simulink model "aocs_plant_pre_high_accuracy_eci_ecef"  (R2025a)
settings: Solver=ode45  StartTime=0  StopTime=200  RelTol=1e-09  AbsTol=1e-10
undefined symbols (not defined in the file): AOCS, AOCS_Config, AOCS_EnvironmentConfig, AOCS_OrbitConfig, IAU, juliandate
libraries: aerolibtransform2 x3, matrix_library x1
settings Model: Creator=juliankazmierski  LastModifiedBy=juliankazmierski

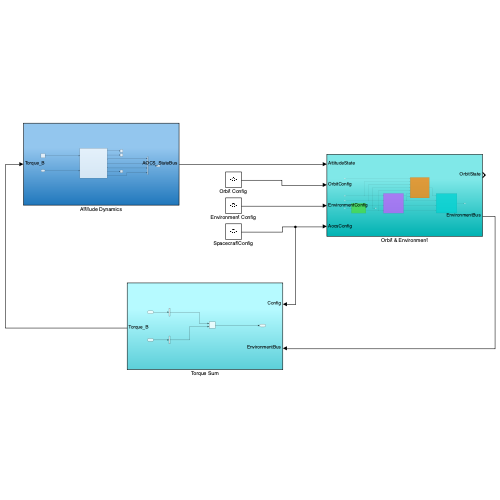
[thumbnail: Simulink's stored preview of the top-level diagram]
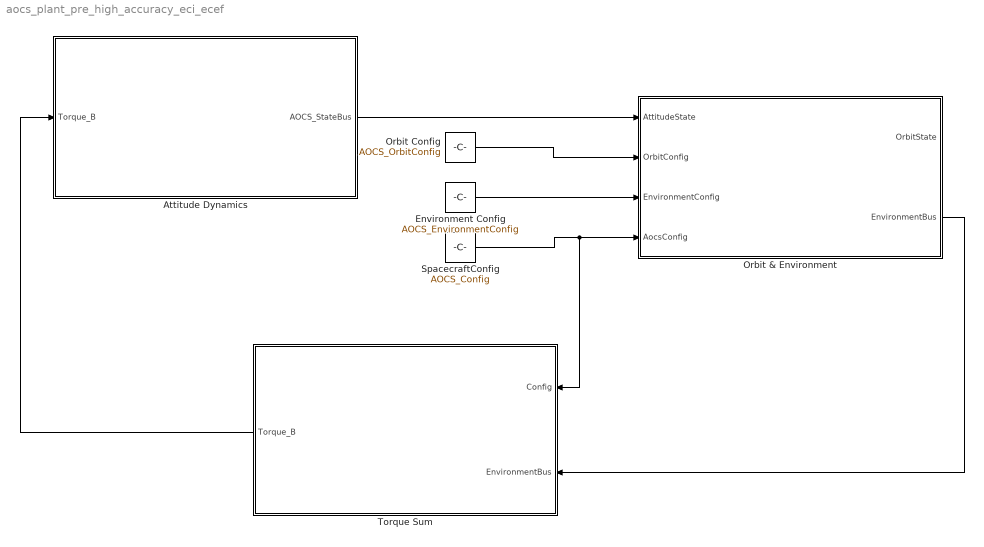
== system aocs_plant_pre_high_accuracy_eci_ecef ==
  Attitude Dynamics : Subsystem
  Environment Config : Constant  Value=AOCS_EnvironmentConfig  OutDataTypeStr=Bus: AOCS_EnvironmentConfigBus
  Orbit & Environment : Subsystem
  Orbit Config : Constant  Value=AOCS_OrbitConfig  VectorParams1D=off  OutDataTypeStr=Bus: AOCS_OrbitConfigBus
  SpacecraftConfig : Constant  Value=AOCS_Config  OutDataTypeStr=Bus: AOCS_ConfigBus
  Torque Sum : Subsystem
  wires:
  SpacecraftConfig/1 -> Orbit & Environment/4(AocsConfig), Torque Sum/1(Config)
  Attitude Dynamics/1(AOCS_StateBus) -> Orbit & Environment/1(AttitudeState)
  Orbit Config/1 -> Orbit & Environment/2(OrbitConfig)
  Environment Config/1 -> Orbit & Environment/3(EnvironmentConfig)
  Orbit & Environment/2(EnvironmentBus) -> Torque Sum/2(EnvironmentBus)
  Torque Sum/1(Torque_B) -> Attitude Dynamics/1(Torque_B)

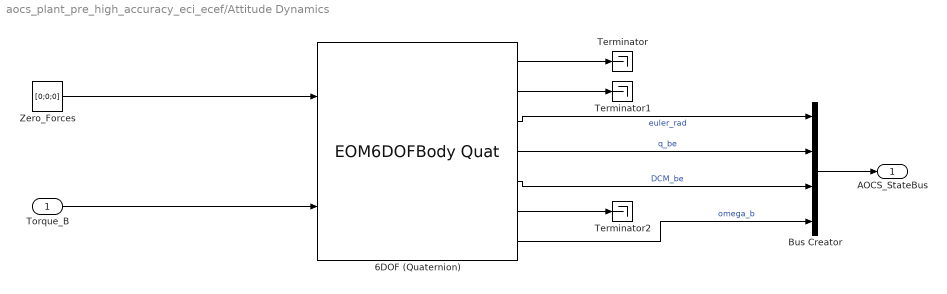
== system aocs_plant_pre_high_accuracy_eci_ecef/Attitude Dynamics ==
  Torque_B : Inport
  6DOF (Quaternion) : EOM6DOFBodyQuat  eul_0=AOCS_Config.euler_BI_0_rad  pm_0=AOCS_Config.omega_BI_B_0  mass_0=3.71  inertia=AOCS_Config.I_B
  Bus Creator : BusCreator  Inputs=4
  Terminator : Terminator
  Terminator1 : Terminator
  Terminator2 : Terminator
  Zero_Forces : Constant  Value=[0;0;0]
  AOCS_StateBus : Outport  OutDataTypeStr=Bus: AOCS_StateBus
  wires:
  Torque_B/1 -> 6DOF (Quaternion)/2
  Zero_Forces/1 -> 6DOF (Quaternion)/1
  6DOF (Quaternion)/1 -> Terminator/1
  6DOF (Quaternion)/2 -> Terminator1/1
  6DOF (Quaternion)/6 -> Terminator2/1
  6DOF (Quaternion)/3 -> Bus Creator/1  "euler_rad"
  6DOF (Quaternion)/5 -> Bus Creator/3  "DCM_be"
  6DOF (Quaternion)/7 -> Bus Creator/4  "omega_b"
  Bus Creator/1 -> AOCS_StateBus/1
  6DOF (Quaternion)/4 -> Bus Creator/2  "q_be"

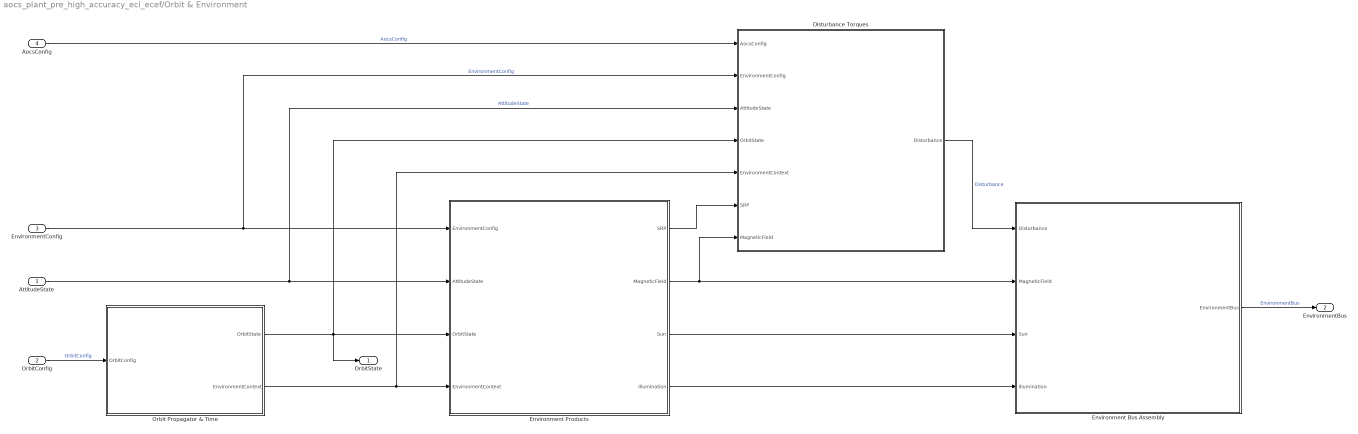
== system aocs_plant_pre_high_accuracy_eci_ecef/Orbit & Environment ==
  AttitudeState : Inport
  OrbitConfig : Inport  Port=2
  EnvironmentConfig : Inport  Port=3
  AocsConfig : Inport  Port=4
  Disturbance Torques : Subsystem
  Environment Bus Assembly : Subsystem
  Environment Products : Subsystem
  Orbit Propagator & Time : Subsystem
  OrbitState : Outport  OutDataTypeStr=Bus: AOCS_OrbitStateBus
  EnvironmentBus : Outport  Port=2  OutDataTypeStr=Bus: AOCS_EnvironmentBus
  wires:
  AocsConfig/1 -> Disturbance Torques/1(AocsConfig)  "AocsConfig"
  Disturbance Torques/1(Disturbance) -> Environment Bus Assembly/1(Disturbance)  "Disturbance"
  Environment Bus Assembly/1(EnvironmentBus) -> EnvironmentBus/1  "EnvironmentBus"
  Environment Products/2(MagneticField) -> Disturbance Torques/7(MagneticField), Environment Bus Assembly/2(MagneticField)
  AttitudeState/1 -> Disturbance Torques/3(AttitudeState), Environment Products/2(AttitudeState)  "AttitudeState"
  Orbit Propagator & Time/1(OrbitState) -> OrbitState/1, Disturbance Torques/4(OrbitState), Environment Products/3(OrbitState)
  Orbit Propagator & Time/2(EnvironmentContext) -> Disturbance Torques/5(EnvironmentContext), Environment Products/4(EnvironmentContext)
  EnvironmentConfig/1 -> Environment Products/1(EnvironmentConfig), Disturbance Torques/2(EnvironmentConfig)  "EnvironmentConfig"
  Environment Products/1(SRP) -> Disturbance Torques/6(SRP)
  Environment Products/4(Illumination) -> Environment Bus Assembly/4(Illumination)
  Environment Products/3(Sun) -> Environment Bus Assembly/3(Sun)
  OrbitConfig/1 -> Orbit Propagator & Time/1(OrbitConfig)  "OrbitConfig"

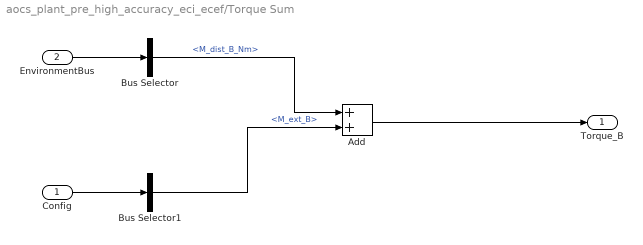
== system aocs_plant_pre_high_accuracy_eci_ecef/Torque Sum ==
  Config : Inport
  EnvironmentBus : Inport  Port=2
  Add : Sum
  Bus Selector : BusSelector  OutputSignals=M_dist_B_Nm
  Bus Selector1 : BusSelector  OutputSignals=M_ext_B
  Torque_B : Outport
  wires:
  EnvironmentBus/1 -> Bus Selector/1
  Bus Selector/1 -> Add/1  "<M_dist_B_Nm>"
  Add/1 -> Torque_B/1
  Config/1 -> Bus Selector1/1
  Bus Selector1/1 -> Add/2  "<M_ext_B>"

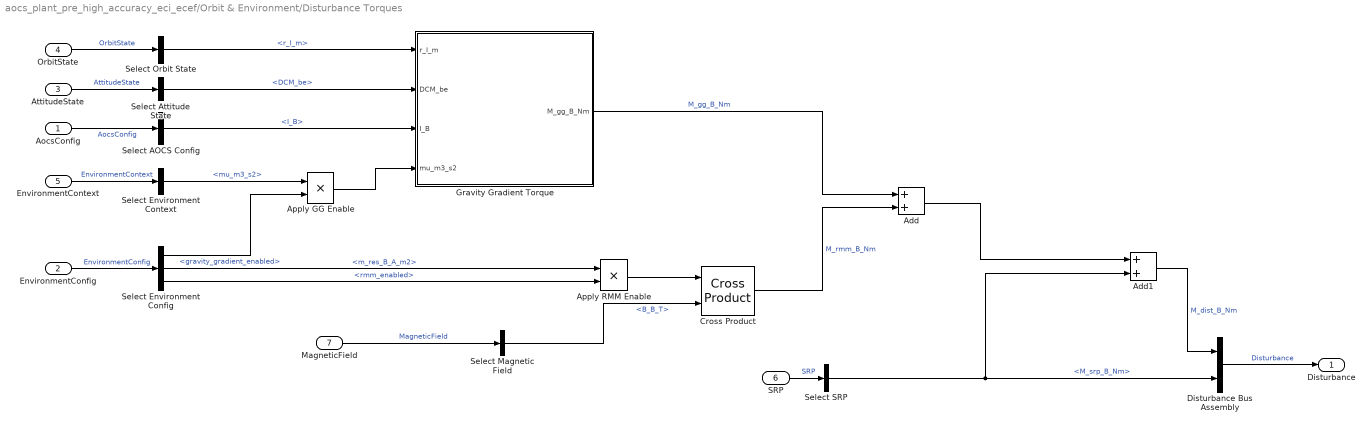
== system aocs_plant_pre_high_accuracy_eci_ecef/Orbit & Environment/Disturbance Torques ==
  AocsConfig : Inport
  EnvironmentConfig : Inport  Port=2
  AttitudeState : Inport  Port=3
  OrbitState : Inport  Port=4
  EnvironmentContext : Inport  Port=5
  SRP : Inport  Port=6
  MagneticField : Inport  Port=7
  Add : Sum
  Add1 : Sum
  Apply GG Enable : Product
  Apply RMM Enable : Product
  Cross Product : matrix_library/Cross Product
  Disturbance Bus Assembly : BusCreator  Inputs=2  OutDataTypeStr=Bus: AOCS_DisturbanceBus
  Gravity Gradient Torque : MATLAB Function  TreatAsAtomicUnit=on
  Select AOCS Config : BusSelector  OutputSignals=I_B
  Select Attitude State : BusSelector  OutputSignals=DCM_be
  Select Environment Config : BusSelector  OutputSignals=gravity_gradient_enabled,m_res_B_A_m2,rmm_enabled
  Select Environment Context : BusSelector  OutputSignals=mu_m3_s2
  Select Magnetic Field : BusSelector  OutputSignals=B_B_T
  Select Orbit State : BusSelector  OutputSignals=r_I_m
  Select SRP : BusSelector  OutputSignals=M_srp_B_Nm
  Disturbance : Outport
  wires:
  Cross Product/1 -> Add/2  "M_rmm_B_Nm"
  Gravity Gradient Torque/1(M_gg_B_Nm) -> Add/1  "M_gg_B_Nm"
  SRP/1 -> Select SRP/1  "SRP"
  Add1/1 -> Disturbance Bus Assembly/1  "M_dist_B_Nm"
  Apply RMM Enable/1 -> Cross Product/1
  Apply GG Enable/1 -> Gravity Gradient Torque/4(mu_m3_s2)
  AocsConfig/1 -> Select AOCS Config/1  "AocsConfig"
  Select AOCS Config/1 -> Gravity Gradient Torque/3(I_B)  "<I_B>"
  EnvironmentConfig/1 -> Select Environment Config/1  "EnvironmentConfig"
  Select Environment Config/2 -> Apply RMM Enable/1  "<m_res_B_A_m2>"
  Select Environment Config/3 -> Apply RMM Enable/2  "<rmm_enabled>"
  Select Environment Config/1 -> Apply GG Enable/2  "<gravity_gradient_enabled>"
  AttitudeState/1 -> Select Attitude State/1  "AttitudeState"
  Select Attitude State/1 -> Gravity Gradient Torque/2(DCM_be)  "<DCM_be>"
  MagneticField/1 -> Select Magnetic Field/1  "MagneticField"
  Select Magnetic Field/1 -> Cross Product/2  "<B_B_T>"
  OrbitState/1 -> Select Orbit State/1  "OrbitState"
  Select Orbit State/1 -> Gravity Gradient Torque/1(r_I_m)  "<r_I_m>"
  EnvironmentContext/1 -> Select Environment Context/1  "EnvironmentContext"
  Select Environment Context/1 -> Apply GG Enable/1  "<mu_m3_s2>"
  Select SRP/1 -> Add1/2, Disturbance Bus Assembly/2  "<M_srp_B_Nm>"
  Disturbance Bus Assembly/1 -> Disturbance/1  "Disturbance"
  Add/1 -> Add1/1

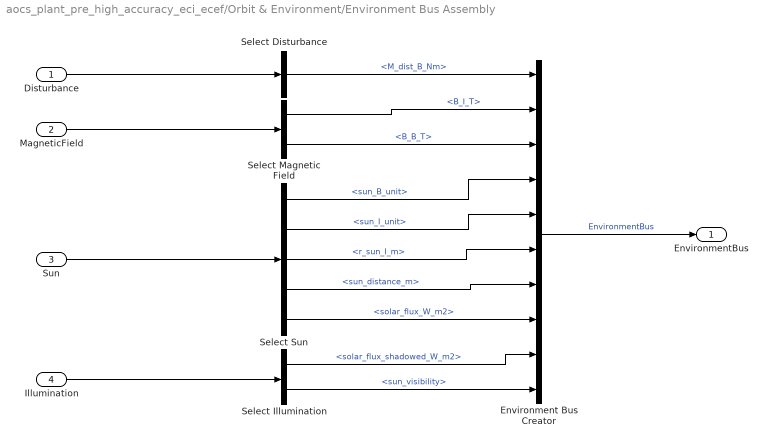
== system aocs_plant_pre_high_accuracy_eci_ecef/Orbit & Environment/Environment Bus Assembly ==
  Disturbance : Inport
  MagneticField : Inport  Port=2
  Sun : Inport  Port=3
  Illumination : Inport  Port=4
  Environment Bus Creator : BusCreator  Inputs=10  OutDataTypeStr=Bus: AOCS_EnvironmentBus
  Select Disturbance : BusSelector  OutputSignals=M_dist_B_Nm
  Select Illumination : BusSelector  OutputSignals=solar_flux_shadowed_W_m2,sun_visibility
  Select Magnetic Field : BusSelector  OutputSignals=B_I_T,B_B_T
  Select Sun : BusSelector  OutputSignals=sun_B_unit,sun_I_unit,r_sun_I_m,sun_distance_m,solar_flux_W_m2
  EnvironmentBus : Outport
  wires:
  Disturbance/1 -> Select Disturbance/1
  Select Disturbance/1 -> Environment Bus Creator/1  "<M_dist_B_Nm>"
  MagneticField/1 -> Select Magnetic Field/1
  Select Magnetic Field/1 -> Environment Bus Creator/2  "<B_I_T>"
  Select Magnetic Field/2 -> Environment Bus Creator/3  "<B_B_T>"
  Sun/1 -> Select Sun/1
  Select Sun/1 -> Environment Bus Creator/4  "<sun_B_unit>"
  Select Sun/2 -> Environment Bus Creator/5  "<sun_I_unit>"
  Select Sun/3 -> Environment Bus Creator/6  "<r_sun_I_m>"
  Select Sun/4 -> Environment Bus Creator/7  "<sun_distance_m>"
  Select Sun/5 -> Environment Bus Creator/8  "<solar_flux_W_m2>"
  Illumination/1 -> Select Illumination/1
  Select Illumination/1 -> Environment Bus Creator/9  "<solar_flux_shadowed_W_m2>"
  Select Illumination/2 -> Environment Bus Creator/10  "<sun_visibility>"
  Environment Bus Creator/1 -> EnvironmentBus/1  "EnvironmentBus"

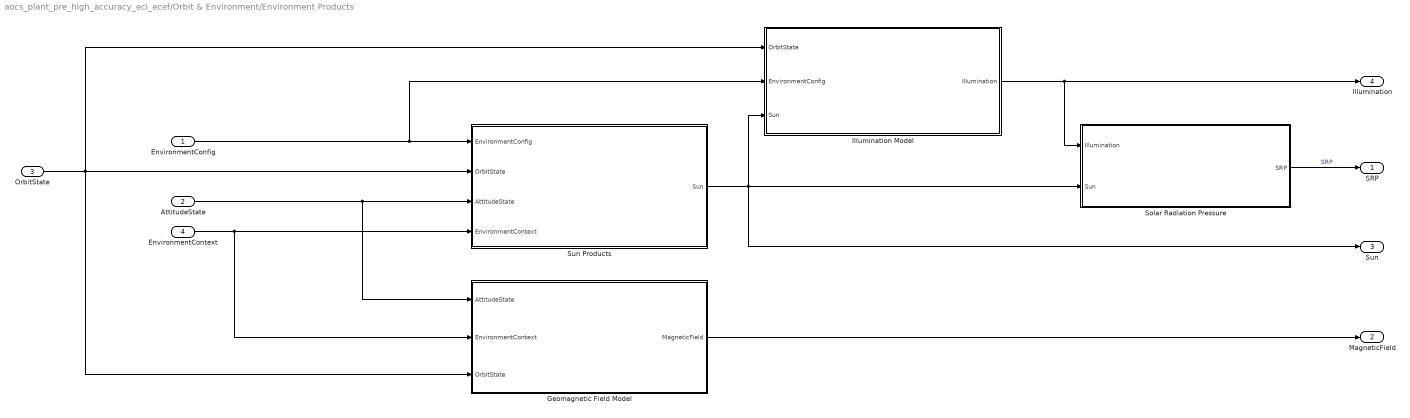
== system aocs_plant_pre_high_accuracy_eci_ecef/Orbit & Environment/Environment Products ==
  EnvironmentConfig : Inport
  AttitudeState : Inport  Port=2
  OrbitState : Inport  Port=3
  EnvironmentContext : Inport  Port=4
  Geomagnetic Field Model : Subsystem
  Illumination Model : Subsystem
  Solar Radiation Pressure : Subsystem
  Sun Products : Subsystem
  SRP : Outport
  MagneticField : Outport  Port=2
  Sun : Outport  Port=3
  Illumination : Outport  Port=4
  wires:
  Sun Products/1(Sun) -> Illumination Model/3(Sun), Solar Radiation Pressure/2(Sun), Sun/1
  Geomagnetic Field Model/1(MagneticField) -> MagneticField/1
  Solar Radiation Pressure/1(SRP) -> SRP/1  "SRP"
  OrbitState/1 -> Geomagnetic Field Model/3(OrbitState), Sun Products/2(OrbitState), Illumination Model/1(OrbitState)
  Illumination Model/1(Illumination) -> Illumination/1, Solar Radiation Pressure/1(Illumination)
  EnvironmentConfig/1 -> Sun Products/1(EnvironmentConfig), Illumination Model/2(EnvironmentConfig)
  EnvironmentContext/1 -> Sun Products/4(EnvironmentContext), Geomagnetic Field Model/2(EnvironmentContext)
  AttitudeState/1 -> Geomagnetic Field Model/1(AttitudeState), Sun Products/3(AttitudeState)

== system aocs_plant_pre_high_accuracy_eci_ecef/Orbit & Environment/Orbit Propagator & Time ==
  OrbitConfig : Inport
  Orbit State : Subsystem
  Orbit and Time Context : Subsystem
  OrbitState : Outport
  EnvironmentContext : Outport  Port=2
  wires:
  OrbitConfig/1 -> Orbit and Time Context/1(In1)
  Orbit State/1(OrbitState) -> OrbitState/1  "OrbitState"
  Orbit and Time Context/1(EnvironmentContext) -> EnvironmentContext/1  "EnvironmentContext"

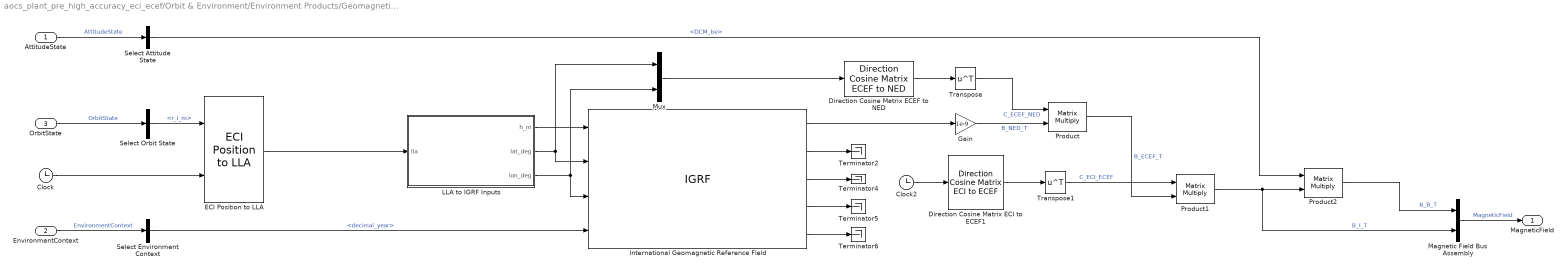
== system aocs_plant_pre_high_accuracy_eci_ecef/Orbit & Environment/Environment Products/Geomagnetic Field Model ==
  AttitudeState : Inport
  EnvironmentContext : Inport  Port=2
  OrbitState : Inport  Port=3
  Clock : Clock
  Clock2 : Clock
  Direction Cosine Matrix ECEF to NED : aerolibtransform2/Direction Cosine Matrix ECEF to NED
  Direction Cosine Matrix ECI to ECEF1 : aerolibtransform2/Direction Cosine Matrix ECI to ECEF  red=IAU-2000/2006  year=2026  month=January  day=1  hour=0  min=0  sec=0  deltaT=Sec  errorflag=Error  extraparamflag=off
      settings: AttributesFormatString=%<red>
  ECI Position to LLA : aerolibtransform2/ECI Position to LLA  red=IAU-2000/2006  year=2026  month=January  day=1  hour=0  min=0  sec=0  deltaT=Sec  errorflag=Error  extraparamflag=off  eunits=Metric (MKS)  earthmodel=WGS84  flat=1/298.257223563  eqradius=6378137
      settings: AttributesFormatString=%<red>
  Gain : Gain  Gain=1e-9
  International Geomagnetic Reference Field : IGRF  month=January  day=1  sv_out=off
      settings: AttributesFormatString=%<generation>
  LLA to IGRF Inputs : MATLAB Function  TreatAsAtomicUnit=on
  Magnetic Field Bus Assembly : BusCreator  Inputs=2  OutDataTypeStr=Bus: AOCS_MagneticFieldBus
  Mux : Mux  Inputs=2
  Product : Product  Multiplication=Matrix(*)
  Product1 : Product  Multiplication=Matrix(*)
  Product2 : Product  Multiplication=Matrix(*)
  Select Attitude State : BusSelector  OutputSignals=DCM_be
  Select Environment Context : BusSelector  OutputSignals=decimal_year
  Select Orbit State : BusSelector  OutputSignals=r_I_m
  Terminator{2,4..6} (4 alike) : Terminator
  Transpose : Math  Operator=transpose
  Transpose1 : Math  Operator=transpose
  MagneticField : Outport
  wires:
  Product2/1 -> Magnetic Field Bus Assembly/1  "B_B_T"
  Product1/1 -> Magnetic Field Bus Assembly/2, Product2/2  "B_I_T"
  Transpose1/1 -> Product1/1  "C_ECI_ECEF"
  Product/1 -> Product1/2  "B_ECEF_T"
  Direction Cosine Matrix ECI to ECEF1/1 -> Transpose1/1
  Transpose/1 -> Product/1  "C_ECEF_NED"
  Gain/1 -> Product/2  "B_NED_T"
  Clock2/1 -> Direction Cosine Matrix ECI to ECEF1/1
  Direction Cosine Matrix ECEF to NED/1 -> Transpose/1
  International Geomagnetic Reference Field/2 -> Terminator2/1
  International Geomagnetic Reference Field/1 -> Gain/1
  Mux/1 -> Direction Cosine Matrix ECEF to NED/1
  International Geomagnetic Reference Field/5 -> Terminator6/1
  LLA to IGRF Inputs/2(lat_deg) -> International Geomagnetic Reference Field/2, Mux/1
  International Geomagnetic Reference Field/4 -> Terminator5/1
  LLA to IGRF Inputs/1(h_m) -> International Geomagnetic Reference Field/1
  LLA to IGRF Inputs/3(lon_deg) -> International Geomagnetic Reference Field/3, Mux/2
  International Geomagnetic Reference Field/3 -> Terminator4/1
  Clock/1 -> ECI Position to LLA/2
  ECI Position to LLA/1 -> LLA to IGRF Inputs/1(lla)
  AttitudeState/1 -> Select Attitude State/1  "AttitudeState"
  Select Attitude State/1 -> Product2/1  "<DCM_be>"
  OrbitState/1 -> Select Orbit State/1  "OrbitState"
  Select Orbit State/1 -> ECI Position to LLA/1  "<r_I_m>"
  EnvironmentContext/1 -> Select Environment Context/1  "EnvironmentContext"
  Select Environment Context/1 -> International Geomagnetic Reference Field/4  "<decimal_year>"
  Magnetic Field Bus Assembly/1 -> MagneticField/1  "MagneticField"

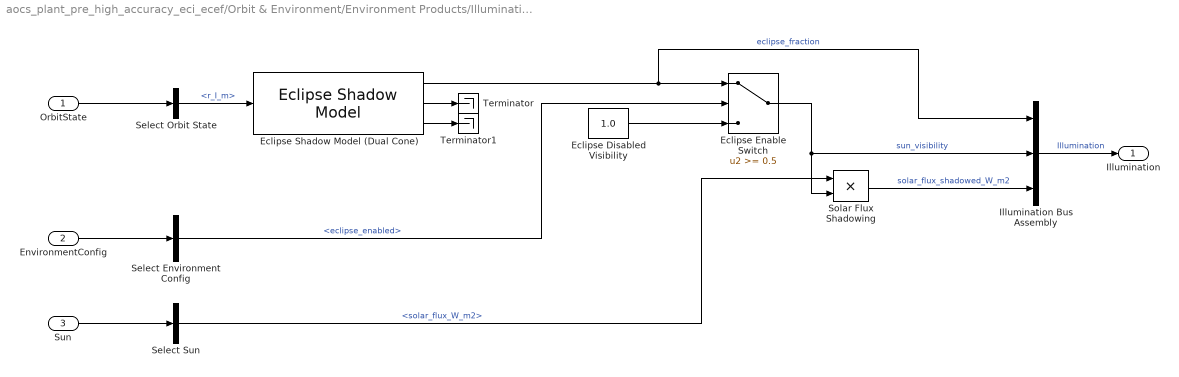
== system aocs_plant_pre_high_accuracy_eci_ecef/Orbit & Environment/Environment Products/Illumination Model ==
  OrbitState : Inport
  EnvironmentConfig : Inport  Port=2
  Sun : Inport  Port=3
  Eclipse Disabled Visibility : Constant  Value=1.0
  Eclipse Enable Switch : Switch  Threshold=0.5  SaturateOnIntegerOverflow=off  InputSameDT=off
  Eclipse Shadow Model (Dual Cone) : EclipseShadowModel  outputShadowRegion=on  startDate=juliandate(2026, 1, 1, 0, 0, 0)  customRadius=6378137  ephemerisStartDate=juliandate(2020, 1, 1, 0, 0, 0)  ephemerisEndDate=juliandate(2030, 1, 1, 0, 0, 0)
  Illumination Bus Assembly : BusCreator  Inputs=3  OutDataTypeStr=Bus: AOCS_IlluminationBus
  Select Environment Config : BusSelector  OutputSignals=eclipse_enabled
  Select Orbit State : BusSelector  OutputSignals=r_I_m
  Select Sun : BusSelector  OutputSignals=solar_flux_W_m2
  Solar Flux Shadowing : Product
  Terminator : Terminator
  Terminator1 : Terminator
  Illumination : Outport
  wires:
  Eclipse Shadow Model (Dual Cone)/2 -> Terminator/1
  Eclipse Shadow Model (Dual Cone)/3 -> Terminator1/1
  Eclipse Shadow Model (Dual Cone)/1 -> Illumination Bus Assembly/1, Eclipse Enable Switch/1  "eclipse_fraction"
  OrbitState/1 -> Select Orbit State/1
  Select Orbit State/1 -> Eclipse Shadow Model (Dual Cone)/1  "<r_I_m>"
  EnvironmentConfig/1 -> Select Environment Config/1
  Select Environment Config/1 -> Eclipse Enable Switch/2  "<eclipse_enabled>"
  Eclipse Disabled Visibility/1 -> Eclipse Enable Switch/3
  Sun/1 -> Select Sun/1
  Select Sun/1 -> Solar Flux Shadowing/1  "<solar_flux_W_m2>"
  Eclipse Enable Switch/1 -> Solar Flux Shadowing/2, Illumination Bus Assembly/2  "sun_visibility"
  Solar Flux Shadowing/1 -> Illumination Bus Assembly/3  "solar_flux_shadowed_W_m2"
  Illumination Bus Assembly/1 -> Illumination/1  "Illumination"

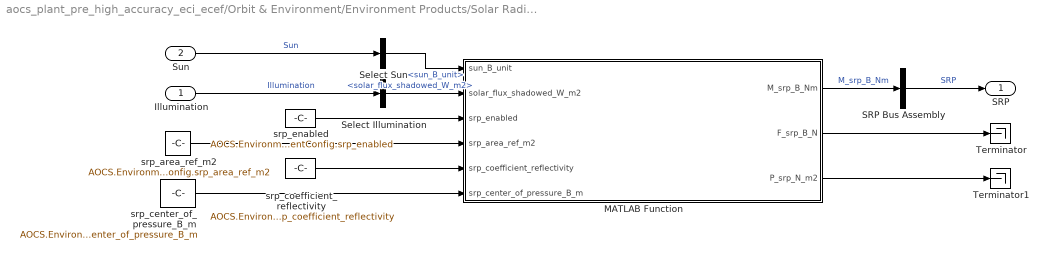
== system aocs_plant_pre_high_accuracy_eci_ecef/Orbit & Environment/Environment Products/Solar Radiation Pressure ==
  Illumination : Inport
  Sun : Inport  Port=2
  MATLAB Function : MATLAB Function  TreatAsAtomicUnit=on
  SRP Bus Assembly : BusCreator  Inputs=1  OutDataTypeStr=Bus: AOCS_SrpBus
  Select Illumination : BusSelector  OutputSignals=solar_flux_shadowed_W_m2
  Select Sun : BusSelector  OutputSignals=sun_B_unit
  Terminator : Terminator
  Terminator1 : Terminator
  srp_area_ref_m2 : Constant  Value=AOCS.EnvironmentConfig.srp_area_ref_m2  VectorParams1D=off  OutDataTypeStr=double
  srp_center_of_pressure_B_m : Constant  Value=AOCS.EnvironmentConfig.srp_center_of_pressure_B_m  VectorParams1D=off  OutDataTypeStr=double
  srp_coefficient_reflectivity : Constant  Value=AOCS.EnvironmentConfig.srp_coefficient_reflectivity  VectorParams1D=off  OutDataTypeStr=double
  srp_enabled : Constant  Value=AOCS.EnvironmentConfig.srp_enabled  VectorParams1D=off  OutDataTypeStr=double
  SRP : Outport
  wires:
  srp_enabled/1 -> MATLAB Function/3(srp_enabled)
  srp_area_ref_m2/1 -> MATLAB Function/4(srp_area_ref_m2)
  srp_coefficient_reflectivity/1 -> MATLAB Function/5(srp_coefficient_reflectivity)
  srp_center_of_pressure_B_m/1 -> MATLAB Function/6(srp_center_of_pressure_B_m)
  MATLAB Function/1(M_srp_B_Nm) -> SRP Bus Assembly/1  "M_srp_B_Nm"
  MATLAB Function/2(F_srp_B_N) -> Terminator/1
  MATLAB Function/3(P_srp_N_m2) -> Terminator1/1
  Sun/1 -> Select Sun/1  "Sun"
  Select Sun/1 -> MATLAB Function/1(sun_B_unit)  "<sun_B_unit>"
  Illumination/1 -> Select Illumination/1  "Illumination"
  Select Illumination/1 -> MATLAB Function/2(solar_flux_shadowed_W_m2)  "<solar_flux_shadowed_W_m2>"
  SRP Bus Assembly/1 -> SRP/1  "SRP"

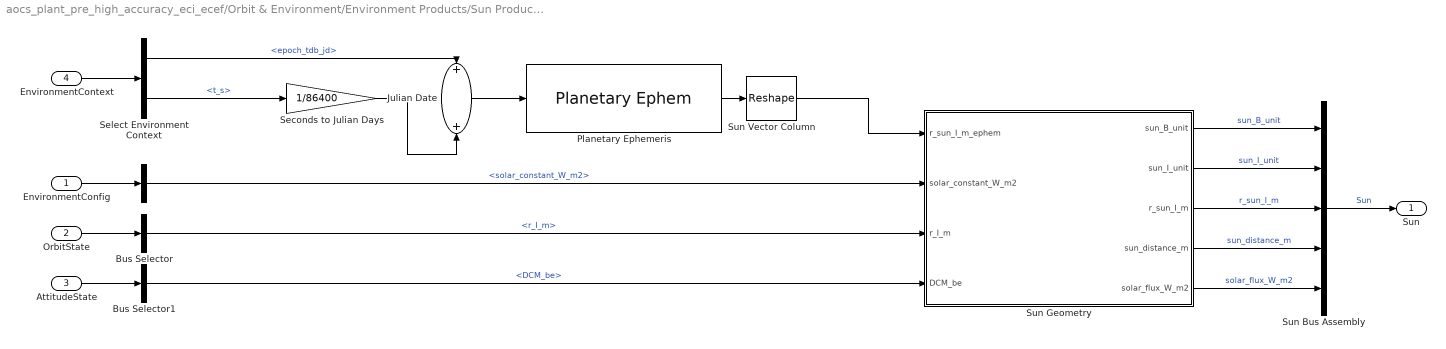
== system aocs_plant_pre_high_accuracy_eci_ecef/Orbit & Environment/Environment Products/Sun Products ==
  EnvironmentConfig : Inport
  OrbitState : Inport  Port=2
  AttitudeState : Inport  Port=3
  EnvironmentContext : Inport  Port=4
  "  " : BusSelector  OutputSignals=solar_constant_W_m2
  Bus Selector : BusSelector  OutputSignals=r_I_m
  Bus Selector1 : BusSelector  OutputSignals=DCM_be
  Julian Date : Sum
  Planetary Ephemeris : PlanetaryEphem  units=m,m/s  target=Sun  useDateRange=on  startDate=juliandate(2020, 1, 1, 0, 0, 0)  endDate=juliandate(2030, 1, 1, 0, 0, 0)  outputVelocity=off
  Seconds to Julian Days : Gain  Gain=1/86400
  Select Environment Context : BusSelector  OutputSignals=epoch_tdb_jd,t_s
  Sun Bus Assembly : BusCreator  Inputs=5  OutDataTypeStr=Bus: AOCS_SunBus
  Sun Geometry : MATLAB Function  TreatAsAtomicUnit=on
  Sun Vector Column : Reshape  OutputDimensionality=Customize  OutputDimensions=[3 1]
  Sun : Outport
  wires:
  EnvironmentContext/1 -> Select Environment Context/1
  Seconds to Julian Days/1 -> Julian Date/2
  Julian Date/1 -> Planetary Ephemeris/1
  Sun Geometry/1(sun_B_unit) -> Sun Bus Assembly/1  "sun_B_unit"
  Sun Geometry/2(sun_I_unit) -> Sun Bus Assembly/2  "sun_I_unit"
  Sun Geometry/3(r_sun_I_m) -> Sun Bus Assembly/3  "r_sun_I_m"
  Sun Geometry/4(sun_distance_m) -> Sun Bus Assembly/4  "sun_distance_m"
  Sun Geometry/5(solar_flux_W_m2) -> Sun Bus Assembly/5  "solar_flux_W_m2"
  Planetary Ephemeris/1 -> Sun Vector Column/1
  Sun Vector Column/1 -> Sun Geometry/1(r_sun_I_m_ephem)
  Select Environment Context/2 -> Seconds to Julian Days/1  "<t_s>"
  Select Environment Context/1 -> Julian Date/1  "<epoch_tdb_jd>"
  EnvironmentConfig/1 -> "  "/1
  "  "/1 -> Sun Geometry/2(solar_constant_W_m2)  "<solar_constant_W_m2>"
  OrbitState/1 -> Bus Selector/1
  Bus Selector/1 -> Sun Geometry/3(r_I_m)  "<r_I_m>"
  AttitudeState/1 -> Bus Selector1/1
  Bus Selector1/1 -> Sun Geometry/4(DCM_be)  "<DCM_be>"
  Sun Bus Assembly/1 -> Sun/1  "Sun"

== system aocs_plant_pre_high_accuracy_eci_ecef/Orbit & Environment/Orbit Propagator & Time/Orbit State ==
  Orbit Propagator : Subsystem
  OrbitState : Outport
  wires:
  Orbit Propagator/1(OrbitState) -> OrbitState/1

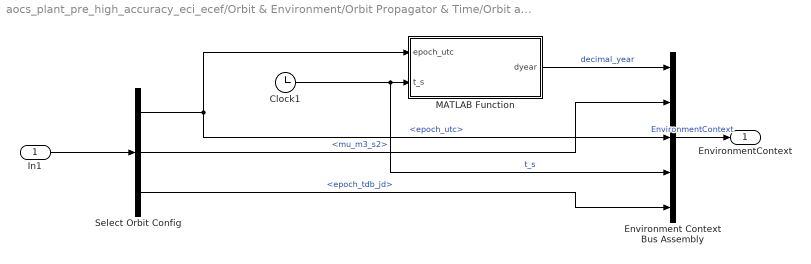
== system aocs_plant_pre_high_accuracy_eci_ecef/Orbit & Environment/Orbit Propagator & Time/Orbit and Time Context ==
  In1 : Inport
  Clock1 : Clock
  Environment Context Bus Assembly : BusCreator  Inputs=5  OutDataTypeStr=Bus: AOCS_EnvironmentContextBus
  MATLAB Function : MATLAB Function  TreatAsAtomicUnit=on
  Select Orbit Config : BusSelector  OutputSignals=epoch_utc,mu_m3_s2,epoch_tdb_jd
  EnvironmentContext : Outport
  wires:
  Select Orbit Config/2 -> Environment Context Bus Assembly/2  "<mu_m3_s2>"
  MATLAB Function/1(dyear) -> Environment Context Bus Assembly/1  "decimal_year"
  In1/1 -> Select Orbit Config/1
  Clock1/1 -> Environment Context Bus Assembly/4, MATLAB Function/2(t_s)  "t_s"
  Select Orbit Config/3 -> Environment Context Bus Assembly/5  "<epoch_tdb_jd>"
  Environment Context Bus Assembly/1 -> EnvironmentContext/1  "EnvironmentContext"
  Select Orbit Config/1 -> MATLAB Function/1(epoch_utc), Environment Context Bus Assembly/3  "<epoch_utc>"

== system aocs_plant_pre_high_accuracy_eci_ecef/Orbit & Environment/Orbit Propagator & Time/Orbit State/Orbit Propagator ==
  Bus Creator : BusCreator  Inputs=2
  Orbit Propagator Kepler (unperturbed) : OrbitPropagator  startDate=AOCS_OrbitConfig.epoch_utc  semiMajorAxis=AOCS_OrbitConfig.semi_major_axis_m  eccentricity=AOCS_OrbitConfig.eccentricity  inclination=AOCS_OrbitConfig.inclination_rad  raan=AOCS_OrbitConfig.raan_rad  argPeriapsis=AOCS_OrbitConfig.argument_of_periapsis_rad  trueAnomaly=AOCS_OrbitConfig.true_anomaly_rad  inertialPosition=[3649700.0 3308200.0 -4676600.0]  inertialVelocity=[-2750.8 6666.4 2573.4]  fixedPosition=[-4142689.0 -2676864.7 -4669861.6]  fixedVelocity=[1452.7 -6720.7 2568.1]  customR=3396200  customMu=4.305e13  customJ2=1.0826269e-03  customOmega=4.06125949e-3  angleUnits=Radians  timeFormat=Gregorian date
  Terminator : Terminator
  OrbitState : Outport  OutDataTypeStr=Bus: AOCS_OrbitStateBus
  wires:
  Orbit Propagator Kepler (unperturbed)/3 -> Terminator/1
  Bus Creator/1 -> OrbitState/1
  Orbit Propagator Kepler (unperturbed)/1 -> Bus Creator/1  "r_I_m"
  Orbit Propagator Kepler (unperturbed)/2 -> Bus Creator/2  "v_I_m_s"

== matlab function aocs_plant_pre_high_accuracy_eci_ecef/Orbit & Environment/Orbit Propagator & Time/Orbit and Time Context/MATLAB Function ==
  data: epoch_utc input; dyear output; t_s input
function dyear = decimalYearUtc(epoch_utc, t_s)
year = floor(epoch_utc(1));
month = floor(epoch_utc(2));
day = floor(epoch_utc(3));
hour = floor(epoch_utc(4));
minute = floor(epoch_utc(5));
second = epoch_utc(6);

monthStart = [0 31 59 90 120 151 181 212 243 273 304 334];
leap = (mod(year,4)==0 && mod(year,100)~=0) || mod(year,400)==0;

leapOffset = 0;
if leap && month > 2
    leapOffset = 1;
end

secIntoYear = (monthStart(month) + leapOffset + day - 1) * 86400 ...
    + hour * 3600 + minute * 60 + second + t_s;

dyear = year + secIntoYear / ((365 + double(leap)) * 86400);
end

== matlab function aocs_plant_pre_high_accuracy_eci_ecef/Orbit & Environment/Disturbance Torques/Gravity Gradient Torque ==
  data: r_I_m input; M_gg_B_Nm output; DCM_be input; I_B input; mu_m3_s2 input
function M_gg_B_Nm = gravityGradientTorque(r_I_m, DCM_be, I_B, mu_m3_s2)
r_norm_m = norm(r_I_m);

if r_norm_m <= 0
    M_gg_B_Nm = zeros(3,1);
    return;
end

r_hat_I = r_I_m / r_norm_m;
r_hat_B = DCM_be * r_hat_I;

M_gg_B_Nm = 3 * mu_m3_s2 / r_norm_m^3 * cross(r_hat_B, I_B * r_hat_B);
end

== matlab function aocs_plant_pre_high_accuracy_eci_ecef/Orbit & Environment/Environment Products/Sun Products/Sun Geometry ==
  data: r_sun_I_m_ephem input size=[3 1]; sun_B_unit output size=[3 1]; solar_constant_W_m2 input size=1; r_I_m input size=[3 1]; DCM_be input size=[3 3]; sun_I_unit output size=[3 1]; r_sun_I_m output size=[3 1]; sun_distance_m output size=1; solar_flux_W_m2 output size=1
function [sun_B_unit, sun_I_unit, r_sun_I_m, sun_distance_m, solar_flux_W_m2] = sunProducts(r_sun_I_m_ephem, solar_constant_W_m2, r_I_m, DCM_be)
%#codegen
sun_B_unit = zeros(3, 1);
sun_I_unit = zeros(3, 1);
r_sun_I_m = zeros(3, 1);
sun_distance_m = 0.0;
solar_flux_W_m2 = 0.0;
[sun_B_unit, sun_I_unit, r_sun_I_m, sun_distance_m, solar_flux_W_m2] = ...
 computeSunProducts(r_sun_I_m_ephem, solar_constant_W_m2, r_I_m, DCM_be);
end

== matlab function aocs_plant_pre_high_accuracy_eci_ecef/Orbit & Environment/Environment Products/Solar Radiation Pressure/MATLAB Function ==
  data: sun_B_unit input size=[3 1]; M_srp_B_Nm output size=[3 1]; solar_flux_shadowed_W_m2 input size=1; srp_enabled input size=1; srp_area_ref_m2 input size=1; srp_coefficient_reflectivity input size=1; srp_center_of_pressure_B_m input size=[3 1]; F_srp_B_N output size=[3 1]; P_srp_N_m2 output size=1
function [M_srp_B_Nm, F_srp_B_N, P_srp_N_m2] = fcn(sun_B_unit, solar_flux_shadowed_W_m2, srp_enabled, srp_area_ref_m2, srp_coefficient_reflectivity, srp_center_of_pressure_B_m)
%#codegen

[M_srp_B_Nm, F_srp_B_N, P_srp_N_m2] = computeSrpTorque( ...
 sun_B_unit, solar_flux_shadowed_W_m2, srp_enabled, ...
 srp_area_ref_m2, srp_coefficient_reflectivity, srp_center_of_pressure_B_m);
end

== matlab function aocs_plant_pre_high_accuracy_eci_ecef/Orbit & Environment/Environment Products/Geomagnetic Field Model/LLA to IGRF Inputs ==
  data: lla input; h_m output; lat_deg output; lon_deg output
function [h_m, lat_deg, lon_deg] = llaToIgrfInputs(lla)
lat_deg = lla(1);
lon_deg = lla(2);
h_m = lla(3);
end
